simulink model "test_mdl_NI"  (R2018a)
settings: Solver=VariableStepAuto  StartTime=0.0  StopTime=10.0  RelTol=1e-3
(part 6 of 24)

== system test_mdl_NI/CAN_Signal/ECM_DIESEL PCM PCM_HEV/PowertrainData_9_0x44C ==
  in : Inport
  AutoTowActv_B_Stat : Subsystem
  AutoTowAllw_D_StatMnu : Subsystem
  GrossTrainWeight_M_Est : Subsystem
  TrailCtlPt_B_Falt : Subsystem
  Veh_V_DsplyTrailCtlSet : Subsystem
  WakeAlarm1_B_Typ : Subsystem
  WakeAlarm1_T_Rq : Subsystem
  bus_creator : BusCreator  Inputs=7
  bus_selector : BusSelector  OutputSignals=GrossTrainWeight_M_Est,AutoTowAllw_D_StatMnu,AutoTowActv_B_Stat,TrailCtlPt_B_Falt,Veh_V_DsplyTrailCtlSet,WakeAlarm1_T_Rq,WakeAlarm1_B_Typ
  out_port : Outport
  wires:
  bus_creator/1 -> out_port/1  "PowertrainData_9_0x44C"
  GrossTrainWeight_M_Est/1(out) -> bus_creator/1  "GrossTrainWeight_M_Est"
  AutoTowAllw_D_StatMnu/1(out) -> bus_creator/2  "AutoTowAllw_D_StatMnu"
  AutoTowActv_B_Stat/1(out) -> bus_creator/3  "AutoTowActv_B_Stat"
  TrailCtlPt_B_Falt/1(out) -> bus_creator/4  "TrailCtlPt_B_Falt"
  Veh_V_DsplyTrailCtlSet/1(out) -> bus_creator/5  "Veh_V_DsplyTrailCtlSet"
  WakeAlarm1_T_Rq/1(out) -> bus_creator/6  "WakeAlarm1_T_Rq"
  WakeAlarm1_B_Typ/1(out) -> bus_creator/7  "WakeAlarm1_B_Typ"
  bus_selector/1 -> GrossTrainWeight_M_Est/1(in)  "<GrossTrainWeight_M_Est>"
  bus_selector/2 -> AutoTowAllw_D_StatMnu/1(in)  "<AutoTowAllw_D_StatMnu>"
  bus_selector/3 -> AutoTowActv_B_Stat/1(in)  "<AutoTowActv_B_Stat>"
  bus_selector/4 -> TrailCtlPt_B_Falt/1(in)  "<TrailCtlPt_B_Falt>"
  bus_selector/5 -> Veh_V_DsplyTrailCtlSet/1(in)  "<Veh_V_DsplyTrailCtlSet>"
  bus_selector/6 -> WakeAlarm1_T_Rq/1(in)  "<WakeAlarm1_T_Rq>"
  bus_selector/7 -> WakeAlarm1_B_Typ/1(in)  "<WakeAlarm1_B_Typ>"
  in/1 -> bus_selector/1

== system test_mdl_NI/CAN_Signal/ECM_DIESEL PCM PCM_HEV/Powertrain_Data_4_0x424 ==
  in : Inport
  BpedDrvMsgTxt_B_Dsply : Subsystem
  FuelLvlWarn_D_ActlEng : Subsystem
  FuelLvl_Pc_DsplyEng : Subsystem
  FuelRange_L_DsplyEng : Subsystem
  RearDiffOilTeWarn_B_Rq : Subsystem
  RearDiffOil_Te_Actl : Subsystem
  SelDrvMdePt_D_Stat : Subsystem
  bus_creator : BusCreator  Inputs=7
  bus_selector : BusSelector  OutputSignals=BpedDrvMsgTxt_B_Dsply,RearDiffOil_Te_Actl,RearDiffOilTeWarn_B_Rq,FuelLvlWarn_D_ActlEng,SelDrvMdePt_D_Stat,FuelRange_L_DsplyEng,FuelLvl_Pc_DsplyEng
  out_port : Outport
  wires:
  bus_creator/1 -> out_port/1  "Powertrain_Data_4_0x424"
  BpedDrvMsgTxt_B_Dsply/1(out) -> bus_creator/1  "BpedDrvMsgTxt_B_Dsply"
  RearDiffOil_Te_Actl/1(out) -> bus_creator/2  "RearDiffOil_Te_Actl"
  RearDiffOilTeWarn_B_Rq/1(out) -> bus_creator/3  "RearDiffOilTeWarn_B_Rq"
  FuelLvlWarn_D_ActlEng/1(out) -> bus_creator/4  "FuelLvlWarn_D_ActlEng"
  SelDrvMdePt_D_Stat/1(out) -> bus_creator/5  "SelDrvMdePt_D_Stat"
  FuelRange_L_DsplyEng/1(out) -> bus_creator/6  "FuelRange_L_DsplyEng"
  FuelLvl_Pc_DsplyEng/1(out) -> bus_creator/7  "FuelLvl_Pc_DsplyEng"
  bus_selector/1 -> BpedDrvMsgTxt_B_Dsply/1(in)  "<BpedDrvMsgTxt_B_Dsply>"
  bus_selector/2 -> RearDiffOil_Te_Actl/1(in)  "<RearDiffOil_Te_Actl>"
  bus_selector/3 -> RearDiffOilTeWarn_B_Rq/1(in)  "<RearDiffOilTeWarn_B_Rq>"
  bus_selector/4 -> FuelLvlWarn_D_ActlEng/1(in)  "<FuelLvlWarn_D_ActlEng>"
  bus_selector/5 -> SelDrvMdePt_D_Stat/1(in)  "<SelDrvMdePt_D_Stat>"
  bus_selector/6 -> FuelRange_L_DsplyEng/1(in)  "<FuelRange_L_DsplyEng>"
  bus_selector/7 -> FuelLvl_Pc_DsplyEng/1(in)  "<FuelLvl_Pc_DsplyEng>"
  in/1 -> bus_selector/1

== system test_mdl_NI/CAN_Signal/ECM_DIESEL PCM PCM_HEV/Powertrain_Data_5_0x43F ==
  in : Inport
  FapLcActv_B_Stat : Subsystem
  FapLcInhbt_B_Rq : Subsystem
  FapLcMaxGrdAbrt_B_Stat : Subsystem
  FapLcMaxGrdInhbt_B_Stat : Subsystem
  FapLcObstcl_B_Stat : Subsystem
  FapLcPrchgBrk_B_Rq : Subsystem
  FapLcStopHold_B_Rq : Subsystem
  bus_creator : BusCreator  Inputs=7
  bus_selector : BusSelector  OutputSignals=FapLcActv_B_Stat,FapLcMaxGrdAbrt_B_Stat,FapLcMaxGrdInhbt_B_Stat,FapLcObstcl_B_Stat,FapLcPrchgBrk_B_Rq,FapLcStopHold_B_Rq,FapLcInhbt_B_Rq
  out_port : Outport
  wires:
  bus_creator/1 -> out_port/1  "Powertrain_Data_5_0x43F"
  FapLcActv_B_Stat/1(out) -> bus_creator/1  "FapLcActv_B_Stat"
  FapLcMaxGrdAbrt_B_Stat/1(out) -> bus_creator/2  "FapLcMaxGrdAbrt_B_Stat"
  FapLcMaxGrdInhbt_B_Stat/1(out) -> bus_creator/3  "FapLcMaxGrdInhbt_B_Stat"
  FapLcObstcl_B_Stat/1(out) -> bus_creator/4  "FapLcObstcl_B_Stat"
  FapLcPrchgBrk_B_Rq/1(out) -> bus_creator/5  "FapLcPrchgBrk_B_Rq"
  FapLcStopHold_B_Rq/1(out) -> bus_creator/6  "FapLcStopHold_B_Rq"
  FapLcInhbt_B_Rq/1(out) -> bus_creator/7  "FapLcInhbt_B_Rq"
  bus_selector/1 -> FapLcActv_B_Stat/1(in)  "<FapLcActv_B_Stat>"
  bus_selector/2 -> FapLcMaxGrdAbrt_B_Stat/1(in)  "<FapLcMaxGrdAbrt_B_Stat>"
  bus_selector/3 -> FapLcMaxGrdInhbt_B_Stat/1(in)  "<FapLcMaxGrdInhbt_B_Stat>"
  bus_selector/4 -> FapLcObstcl_B_Stat/1(in)  "<FapLcObstcl_B_Stat>"
  bus_selector/5 -> FapLcPrchgBrk_B_Rq/1(in)  "<FapLcPrchgBrk_B_Rq>"
  bus_selector/6 -> FapLcStopHold_B_Rq/1(in)  "<FapLcStopHold_B_Rq>"
  bus_selector/7 -> FapLcInhbt_B_Rq/1(in)  "<FapLcInhbt_B_Rq>"
  in/1 -> bus_selector/1

== system test_mdl_NI/CAN_Signal/ECM_DIESEL PCM PCM_HEV/Stop_Start_0x166 ==
  in : Inport
  AutoStopPtDelta_I_Est : Subsystem
  HiElPwInhbt_B_Stat : Subsystem
  OdoTripVerify_L_Actl : Subsystem
  StopStrtDrvMde_D_Indic : Subsystem
  StopStrtIODTxt_D_Rq : Subsystem
  StopStrtMsgTxt_D_Rq : Subsystem
  StopStrtStdby_D_Indic : Subsystem
  bus_creator : BusCreator  Inputs=7
  bus_selector : BusSelector  OutputSignals=AutoStopPtDelta_I_Est,HiElPwInhbt_B_Stat,StopStrtDrvMde_D_Indic,StopStrtMsgTxt_D_Rq,OdoTripVerify_L_Actl,StopStrtStdby_D_Indic,StopStrtIODTxt_D_Rq
  out_port : Outport
  wires:
  bus_creator/1 -> out_port/1  "Stop_Start_0x166"
  AutoStopPtDelta_I_Est/1(out) -> bus_creator/1  "AutoStopPtDelta_I_Est"
  HiElPwInhbt_B_Stat/1(out) -> bus_creator/2  "HiElPwInhbt_B_Stat"
  StopStrtDrvMde_D_Indic/1(out) -> bus_creator/3  "StopStrtDrvMde_D_Indic"
  StopStrtMsgTxt_D_Rq/1(out) -> bus_creator/4  "StopStrtMsgTxt_D_Rq"
  OdoTripVerify_L_Actl/1(out) -> bus_creator/5  "OdoTripVerify_L_Actl"
  StopStrtStdby_D_Indic/1(out) -> bus_creator/6  "StopStrtStdby_D_Indic"
  StopStrtIODTxt_D_Rq/1(out) -> bus_creator/7  "StopStrtIODTxt_D_Rq"
  bus_selector/1 -> AutoStopPtDelta_I_Est/1(in)  "<AutoStopPtDelta_I_Est>"
  bus_selector/2 -> HiElPwInhbt_B_Stat/1(in)  "<HiElPwInhbt_B_Stat>"
  bus_selector/3 -> StopStrtDrvMde_D_Indic/1(in)  "<StopStrtDrvMde_D_Indic>"
  bus_selector/4 -> StopStrtMsgTxt_D_Rq/1(in)  "<StopStrtMsgTxt_D_Rq>"
  bus_selector/5 -> OdoTripVerify_L_Actl/1(in)  "<OdoTripVerify_L_Actl>"
  bus_selector/6 -> StopStrtStdby_D_Indic/1(in)  "<StopStrtStdby_D_Indic>"
  bus_selector/7 -> StopStrtIODTxt_D_Rq/1(in)  "<StopStrtIODTxt_D_Rq>"
  in/1 -> bus_selector/1

== system test_mdl_NI/CAN_Signal/ECM_DIESEL PCM PCM_HEV/TesterPhysicalResPCM_0x7E8 ==
  in : Inport
  TesterPhysicalResPCM : Subsystem
  bus_creator : BusCreator  Inputs=1
  bus_selector : BusSelector  OutputSignals=TesterPhysicalResPCM
  out_port : Outport
  wires:
  bus_creator/1 -> out_port/1  "TesterPhysicalResPCM_0x7E8"
  TesterPhysicalResPCM/1(out) -> bus_creator/1  "TesterPhysicalResPCM"
  bus_selector/1 -> TesterPhysicalResPCM/1(in)  "<TesterPhysicalResPCM>"
  in/1 -> bus_selector/1

== system test_mdl_NI/CAN_Signal/ECM_DIESEL PCM PCM_HEV/TorqueDataEngFlags_0x200 ==
  in : Inport
  PrplWhlTotTqRq_No_Cnt : Subsystem
  PrplWhlTotTqRq_No_Cs : Subsystem
  PrplWhlTot_Tq_LimMn : Subsystem
  PrplWhlTot_Tq_Rq : Subsystem
  PtDrvMde_D_Stat : Subsystem
  bus_creator : BusCreator  Inputs=5
  bus_selector : BusSelector  OutputSignals=PrplWhlTot_Tq_LimMn,PrplWhlTot_Tq_Rq,PtDrvMde_D_Stat,PrplWhlTotTqRq_No_Cnt,PrplWhlTotTqRq_No_Cs
  out_port : Outport
  wires:
  bus_creator/1 -> out_port/1  "TorqueDataEngFlags_0x200"
  PrplWhlTot_Tq_LimMn/1(out) -> bus_creator/1  "PrplWhlTot_Tq_LimMn"
  PrplWhlTot_Tq_Rq/1(out) -> bus_creator/2  "PrplWhlTot_Tq_Rq"
  PtDrvMde_D_Stat/1(out) -> bus_creator/3  "PtDrvMde_D_Stat"
  PrplWhlTotTqRq_No_Cnt/1(out) -> bus_creator/4  "PrplWhlTotTqRq_No_Cnt"
  PrplWhlTotTqRq_No_Cs/1(out) -> bus_creator/5  "PrplWhlTotTqRq_No_Cs"
  bus_selector/1 -> PrplWhlTot_Tq_LimMn/1(in)  "<PrplWhlTot_Tq_LimMn>"
  bus_selector/2 -> PrplWhlTot_Tq_Rq/1(in)  "<PrplWhlTot_Tq_Rq>"
  bus_selector/3 -> PtDrvMde_D_Stat/1(in)  "<PtDrvMde_D_Stat>"
  bus_selector/4 -> PrplWhlTotTqRq_No_Cnt/1(in)  "<PrplWhlTotTqRq_No_Cnt>"
  bus_selector/5 -> PrplWhlTotTqRq_No_Cs/1(in)  "<PrplWhlTotTqRq_No_Cs>"
  in/1 -> bus_selector/1

== system test_mdl_NI/CAN_Signal/ECM_DIESEL PCM PCM_HEV/TransGearData ==
  in : Inport
  GboxOil_Te_Actl : Subsystem
  GearLvrPos_D_Actl : Subsystem
  SelDrvMdeSwtch_D_Stat3 : Subsystem
  TrnShifActv_B_Actl : Subsystem
  TrnSrvcRqd_B_Rq : Subsystem
  bus_creator : BusCreator  Inputs=5
  bus_selector : BusSelector  OutputSignals=GboxOil_Te_Actl,GearLvrPos_D_Actl,SelDrvMdeSwtch_D_Stat3,TrnShifActv_B_Actl,TrnSrvcRqd_B_Rq
  out_port : Outport
  wires:
  bus_creator/1 -> out_port/1  "TransGearData"
  GboxOil_Te_Actl/1(out) -> bus_creator/1  "GboxOil_Te_Actl"
  GearLvrPos_D_Actl/1(out) -> bus_creator/2  "GearLvrPos_D_Actl"
  SelDrvMdeSwtch_D_Stat3/1(out) -> bus_creator/3  "SelDrvMdeSwtch_D_Stat3"
  TrnShifActv_B_Actl/1(out) -> bus_creator/4  "TrnShifActv_B_Actl"
  TrnSrvcRqd_B_Rq/1(out) -> bus_creator/5  "TrnSrvcRqd_B_Rq"
  bus_selector/1 -> GboxOil_Te_Actl/1(in)  "<GboxOil_Te_Actl>"
  bus_selector/2 -> GearLvrPos_D_Actl/1(in)  "<GearLvrPos_D_Actl>"
  bus_selector/3 -> SelDrvMdeSwtch_D_Stat3/1(in)  "<SelDrvMdeSwtch_D_Stat3>"
  bus_selector/4 -> TrnShifActv_B_Actl/1(in)  "<TrnShifActv_B_Actl>"
  bus_selector/5 -> TrnSrvcRqd_B_Rq/1(in)  "<TrnSrvcRqd_B_Rq>"
  in/1 -> bus_selector/1

== system test_mdl_NI/CAN_Signal/ECM_DIESEL PCM PCM_HEV/VehicleOperatingModes_0x167 ==
  in : Inport
  ElPw_D_Stat : Subsystem
  ElPw_D_StatStrtStop : Subsystem
  Eng_D_Stat : Subsystem
  PlgActvArb_B_Actl : Subsystem
  PrplWhlRgenMn_Tq_Actl : Subsystem
  PrplWhlTot2_Tq_Actl : Subsystem
  PwPckTq_D_Stat : Subsystem
  TrnAinTq_D_Qf : Subsystem
  TrnAin_Tq_Actl : Subsystem
  bus_creator : BusCreator  Inputs=9
  bus_selector : BusSelector  OutputSignals=Eng_D_Stat,PwPckTq_D_Stat,ElPw_D_Stat,PlgActvArb_B_Actl,PrplWhlTot2_Tq_Actl,ElPw_D_StatStrtStop,PrplWhlRgenMn_Tq_Actl,TrnAinTq_D_Qf,TrnAin_Tq_Actl
  out_port : Outport
  wires:
  bus_creator/1 -> out_port/1  "VehicleOperatingModes_0x167"
  Eng_D_Stat/1(out) -> bus_creator/1  "Eng_D_Stat"
  PwPckTq_D_Stat/1(out) -> bus_creator/2  "PwPckTq_D_Stat"
  ElPw_D_Stat/1(out) -> bus_creator/3  "ElPw_D_Stat"
  PlgActvArb_B_Actl/1(out) -> bus_creator/4  "PlgActvArb_B_Actl"
  PrplWhlTot2_Tq_Actl/1(out) -> bus_creator/5  "PrplWhlTot2_Tq_Actl"
  ElPw_D_StatStrtStop/1(out) -> bus_creator/6  "ElPw_D_StatStrtStop"
  PrplWhlRgenMn_Tq_Actl/1(out) -> bus_creator/7  "PrplWhlRgenMn_Tq_Actl"
  TrnAinTq_D_Qf/1(out) -> bus_creator/8  "TrnAinTq_D_Qf"
  TrnAin_Tq_Actl/1(out) -> bus_creator/9  "TrnAin_Tq_Actl"
  bus_selector/1 -> Eng_D_Stat/1(in)  "<Eng_D_Stat>"
  bus_selector/2 -> PwPckTq_D_Stat/1(in)  "<PwPckTq_D_Stat>"
  bus_selector/3 -> ElPw_D_Stat/1(in)  "<ElPw_D_Stat>"
  bus_selector/4 -> PlgActvArb_B_Actl/1(in)  "<PlgActvArb_B_Actl>"
  bus_selector/5 -> PrplWhlTot2_Tq_Actl/1(in)  "<PrplWhlTot2_Tq_Actl>"
  bus_selector/6 -> ElPw_D_StatStrtStop/1(in)  "<ElPw_D_StatStrtStop>"
  bus_selector/7 -> PrplWhlRgenMn_Tq_Actl/1(in)  "<PrplWhlRgenMn_Tq_Actl>"
  bus_selector/8 -> TrnAinTq_D_Qf/1(in)  "<TrnAinTq_D_Qf>"
  bus_selector/9 -> TrnAin_Tq_Actl/1(in)  "<TrnAin_Tq_Actl>"
  in/1 -> bus_selector/1

== system test_mdl_NI/CAN_Signal/GWM/GSM ==
  in : Inport
  Gear_Shift_by_Wire_2_FD1_168 : Subsystem
  Gear_Shift_by_Wire_FD1_5A : Subsystem
  bus_creator : BusCreator  Inputs=2
  bus_selector : BusSelector  OutputSignals=Gear_Shift_by_Wire_2_FD1_168,Gear_Shift_by_Wire_FD1_5A
  out_port : Outport
  wires:
  bus_creator/1 -> out_port/1  "GSM"
  Gear_Shift_by_Wire_2_FD1_168/1(out_port) -> bus_creator/1  "Gear_Shift_by_Wire_2_FD1_168"
  Gear_Shift_by_Wire_FD1_5A/1(out_port) -> bus_creator/2  "Gear_Shift_by_Wire_FD1_5A"
  bus_selector/1 -> Gear_Shift_by_Wire_2_FD1_168/1(in)  "<Gear_Shift_by_Wire_2_FD1_168>"
  bus_selector/2 -> Gear_Shift_by_Wire_FD1_5A/1(in)  "<Gear_Shift_by_Wire_FD1_5A>"
  in/1 -> bus_selector/1

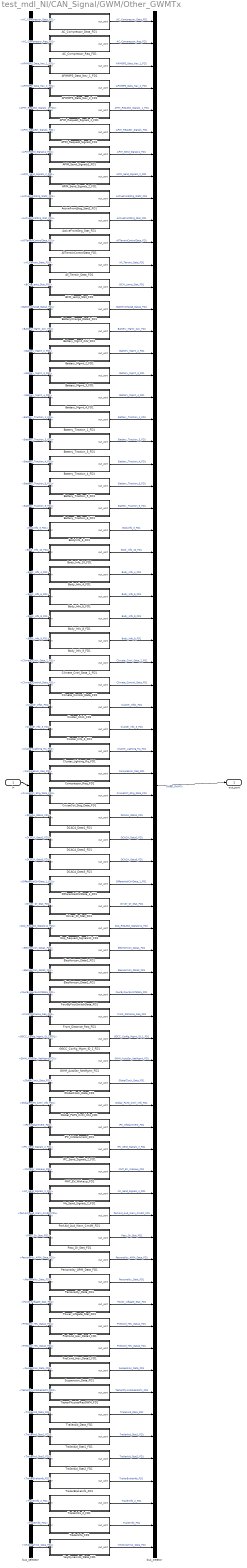
== system test_mdl_NI/CAN_Signal/GWM/Other_GWMTx ==
  in : Inport
  AC_Compressor_Data_FD1 : Subsystem
  AC_Compressor_Req_FD1 : Subsystem
  APIMGPS_Data_Nav_1_FD1 : Subsystem
  APIMGPS_Data_Nav_2_FD1 : Subsystem
  APIM_Request_Signals_1_FD1 : Subsystem
  APIM_Request_Signals_FD1 : Subsystem
  APIM_Send_Signals1_FD1 : Subsystem
  APIM_Send_Signals_2_FD1 : Subsystem
  ActiveFrontStrg_Stat2_FD1 : Subsystem
  ActiveFrontStrg_Stat_FD1 : Subsystem
  AllTerrainControlData_FD1 : Subsystem
  All_Terrain_Data_FD1 : Subsystem
  BCM_Lamp_Stat_FD1 : Subsystem
  BatteryCharge_Data2_FD1 : Subsystem
  Battery_Mgmt_24V_FD1 : Subsystem
  Battery_Mgmt_2_FD1 : Subsystem
  Battery_Mgmt_3_FD1 : Subsystem
  Battery_Mgmt_4_FD1 : Subsystem
  Battery_Traction_1_FD1 : Subsystem
  Battery_Traction_3_FD1 : Subsystem
  Battery_Traction_4_FD1 : Subsystem
  Battery_Traction_5_FD1 : Subsystem
  Battery_Traction_6_FD1 : Subsystem
  BodyInfo_3_FD1 : Subsystem
  Body_Info_10_FD1 : Subsystem
  Body_Info_4_FD1 : Subsystem
  Body_Info_6_FD1 : Subsystem
  Body_Info_8_FD1 : Subsystem
  Body_Info_9_FD1 : Subsystem
  Climate_Cntrl_Data_2_FD1 : Subsystem
  Climate_Control_Data_FD1 : Subsystem
  Cluster_Info1_FD1 : Subsystem
  Cluster_Info_3_FD1 : Subsystem
  Cluster_Lighting_Rq_FD1 : Subsystem
  Compressor_Req_FD1 : Subsystem
  CruiseCtrl_Strg_Data_FD1 : Subsystem
  DCACA_Data1_FD1 : Subsystem
  DCACA_Data2_FD1 : Subsystem
  DCACA_Data3_FD1 : Subsystem
  DifferentialCtrlData_1_FD1 : Subsystem
  Driver_Dr_Stat_FD1 : Subsystem
  Dsp_Request_Signals11_FD1 : Subsystem
  ElecHorizon_Data1_FD1 : Subsystem
  ElecHorizon_Data2_FD1 : Subsystem
  FourByFourSwitchData_FD1 : Subsystem
  Front_Distance_Req_FD1 : Subsystem
  GGCC_Config_Mgmt_ID_1_FD1 : Subsystem
  GWM_AutoSar_NetMgmt_FD1 : Subsystem
  GlobalClock_Data_FD1 : Subsystem
  Global_PATS_Cntrl_Info_FD1 : Subsystem
  IPC_Infotainment_FD1 : Subsystem
  IPC_Send_Signals_2_FD1 : Subsystem
  MHT_EV_Wakeup_FD1 : Subsystem
  Mc_Send_Signals_2_FD1 : Subsystem
  ParkAid_Aud_Warn_CmdM_FD1 : Subsystem
  Pass_Dr_Stat_FD1 : Subsystem
  Personality_APIM_Data_FD1 : Subsystem
  Personality_Data_FD1 : Subsystem
  Power_Liftgate_Stat_FD1 : Subsystem
  PreCond_Hev_Data1_FD1 : Subsystem
  PreCond_Hev_Data2_FD1 : Subsystem
  Suspension_Data_FD1 : Subsystem
  TesterPhysicalResGWM_FD1 : Subsystem
  TrailerAid_Data_FD1 : Subsystem
  TrailerAid_Stat1_FD1 : Subsystem
  TrailerAid_Stat2_FD1 : Subsystem
  TrailerBrakeInfo_FD1 : Subsystem
  TrailerInfo_2_FD1 : Subsystem
  TrailerInfo_FD1 : Subsystem
  VeyDynamics_Data_FD1 : Subsystem
  bus_creator : BusCreator  Inputs=70
  bus_selector : BusSelector  OutputSignals=AC_Compressor_Data_FD1,AC_Compressor_Req_FD1,APIMGPS_Data_Nav_1_FD1,APIMGPS_Data_Nav_2_FD1,APIM_Request_Signals_1_FD1,APIM_Request_Signals_FD1,APIM_Send_Signals1_FD1,APIM_Send_Signals_2_FD1,ActiveFrontStrg_Stat2_FD1,ActiveFrontStrg_Stat_FD1,AllTerrainControlData_FD1,All_Terrain_Data_FD1,BCM_Lamp_Stat_FD1,BatteryCharge_Data2_FD1,Battery_Mgmt_24V_FD1,Battery_Mgmt_2_FD1,Battery_Mgmt_3_FD1,Battery_Mgmt_4_FD1,Battery_Traction_1_FD1,Battery_Traction_3_FD1,Battery_Traction_4_FD1,Battery_Traction_5_FD1,Battery_Traction_6_FD1,BodyInfo_3_FD1,Body_Info_10_FD1,Body_Info_4_FD1,Body_Info_6_FD1,Body_Info_8_FD1,Body_Info_9_FD1,Climate_Cntrl_Data_2_FD1,Climate_Control_Data_FD1,Cluster_Info1_FD1,Cluster_Info_3_FD1,Cluster_Lighting_Rq_FD1,Compressor_Req_FD1,CruiseCtrl_Strg_Data_FD1,DCACA_Data1_FD1,DCACA_Data2_FD1,DCACA_Data3_FD1,DifferentialCtrlData_1_FD1,Driver_Dr_Stat_FD1,Dsp_Request_Signals11_FD1,ElecHorizon_Data1_FD1,ElecHorizon_Data2_FD1,FourByFourSwitchData_FD1,Front_Distance_Req_FD1,GGCC_Config_Mgmt_ID_1_FD1,GWM_AutoSar_NetMgmt_FD1,GlobalClock_Data_FD1,Global_PATS_Cntrl_Info_FD1,IPC_Infotainment_FD1,IPC_Send_Signals_2_FD1,MHT_EV_Wakeup_FD1,Mc_Send_Signals_2_FD1,ParkAid_Aud_Warn_CmdM_FD1,Pass_Dr_Stat_FD1,Personality_APIM_Data_FD1,Personality_Data_FD1,Power_Liftgate_Stat_FD1,PreCond_Hev_Data1_FD1,PreCond_Hev_Data2_FD1,Suspension_Data_FD1,TesterPhysicalResGWM_FD1,TrailerAid_Data_FD1,TrailerAid_Stat1_FD1,TrailerAid_Stat2_FD1,TrailerBrakeInfo_FD1,TrailerInfo_2_FD1,TrailerInfo_FD1,VeyDynamics_Data_FD1
  out_port : Outport
  wires:
  bus_creator/1 -> out_port/1  "Other_GWMTx"
  AC_Compressor_Data_FD1/1(out_port) -> bus_creator/1  "AC_Compressor_Data_FD1"
  AC_Compressor_Req_FD1/1(out_port) -> bus_creator/2  "AC_Compressor_Req_FD1"
  APIMGPS_Data_Nav_1_FD1/1(out_port) -> bus_creator/3  "APIMGPS_Data_Nav_1_FD1"
  APIMGPS_Data_Nav_2_FD1/1(out_port) -> bus_creator/4  "APIMGPS_Data_Nav_2_FD1"
  APIM_Request_Signals_1_FD1/1(out_port) -> bus_creator/5  "APIM_Request_Signals_1_FD1"
  APIM_Request_Signals_FD1/1(out_port) -> bus_creator/6  "APIM_Request_Signals_FD1"
  APIM_Send_Signals1_FD1/1(out_port) -> bus_creator/7  "APIM_Send_Signals1_FD1"
  APIM_Send_Signals_2_FD1/1(out_port) -> bus_creator/8  "APIM_Send_Signals_2_FD1"
  ActiveFrontStrg_Stat2_FD1/1(out_port) -> bus_creator/9  "ActiveFrontStrg_Stat2_FD1"
  ActiveFrontStrg_Stat_FD1/1(out_port) -> bus_creator/10  "ActiveFrontStrg_Stat_FD1"
  AllTerrainControlData_FD1/1(out_port) -> bus_creator/11  "AllTerrainControlData_FD1"
  All_Terrain_Data_FD1/1(out_port) -> bus_creator/12  "All_Terrain_Data_FD1"
  BCM_Lamp_Stat_FD1/1(out_port) -> bus_creator/13  "BCM_Lamp_Stat_FD1"
  BatteryCharge_Data2_FD1/1(out_port) -> bus_creator/14  "BatteryCharge_Data2_FD1"
  Battery_Mgmt_24V_FD1/1(out_port) -> bus_creator/15  "Battery_Mgmt_24V_FD1"
  Battery_Mgmt_2_FD1/1(out_port) -> bus_creator/16  "Battery_Mgmt_2_FD1"
  Battery_Mgmt_3_FD1/1(out_port) -> bus_creator/17  "Battery_Mgmt_3_FD1"
  Battery_Mgmt_4_FD1/1(out_port) -> bus_creator/18  "Battery_Mgmt_4_FD1"
  Battery_Traction_1_FD1/1(out_port) -> bus_creator/19  "Battery_Traction_1_FD1"
  Battery_Traction_3_FD1/1(out_port) -> bus_creator/20  "Battery_Traction_3_FD1"
  Battery_Traction_4_FD1/1(out_port) -> bus_creator/21  "Battery_Traction_4_FD1"
  Battery_Traction_5_FD1/1(out_port) -> bus_creator/22  "Battery_Traction_5_FD1"
  Battery_Traction_6_FD1/1(out_port) -> bus_creator/23  "Battery_Traction_6_FD1"
  BodyInfo_3_FD1/1(out_port) -> bus_creator/24  "BodyInfo_3_FD1"
  Body_Info_10_FD1/1(out_port) -> bus_creator/25  "Body_Info_10_FD1"
  Body_Info_4_FD1/1(out_port) -> bus_creator/26  "Body_Info_4_FD1"
  Body_Info_6_FD1/1(out_port) -> bus_creator/27  "Body_Info_6_FD1"
  Body_Info_8_FD1/1(out_port) -> bus_creator/28  "Body_Info_8_FD1"
  Body_Info_9_FD1/1(out_port) -> bus_creator/29  "Body_Info_9_FD1"
  Climate_Cntrl_Data_2_FD1/1(out_port) -> bus_creator/30  "Climate_Cntrl_Data_2_FD1"
  Climate_Control_Data_FD1/1(out_port) -> bus_creator/31  "Climate_Control_Data_FD1"
  Cluster_Info1_FD1/1(out_port) -> bus_creator/32  "Cluster_Info1_FD1"
  Cluster_Info_3_FD1/1(out_port) -> bus_creator/33  "Cluster_Info_3_FD1"
  Cluster_Lighting_Rq_FD1/1(out_port) -> bus_creator/34  "Cluster_Lighting_Rq_FD1"
  Compressor_Req_FD1/1(out_port) -> bus_creator/35  "Compressor_Req_FD1"
  CruiseCtrl_Strg_Data_FD1/1(out_port) -> bus_creator/36  "CruiseCtrl_Strg_Data_FD1"
  DCACA_Data1_FD1/1(out_port) -> bus_creator/37  "DCACA_Data1_FD1"
  DCACA_Data2_FD1/1(out_port) -> bus_creator/38  "DCACA_Data2_FD1"
  DCACA_Data3_FD1/1(out_port) -> bus_creator/39  "DCACA_Data3_FD1"
  DifferentialCtrlData_1_FD1/1(out_port) -> bus_creator/40  "DifferentialCtrlData_1_FD1"
  Driver_Dr_Stat_FD1/1(out_port) -> bus_creator/41  "Driver_Dr_Stat_FD1"
  Dsp_Request_Signals11_FD1/1(out_port) -> bus_creator/42  "Dsp_Request_Signals11_FD1"
  ElecHorizon_Data1_FD1/1(out_port) -> bus_creator/43  "ElecHorizon_Data1_FD1"
  ElecHorizon_Data2_FD1/1(out_port) -> bus_creator/44  "ElecHorizon_Data2_FD1"
  FourByFourSwitchData_FD1/1(out_port) -> bus_creator/45  "FourByFourSwitchData_FD1"
  Front_Distance_Req_FD1/1(out_port) -> bus_creator/46  "Front_Distance_Req_FD1"
  GGCC_Config_Mgmt_ID_1_FD1/1(out_port) -> bus_creator/47  "GGCC_Config_Mgmt_ID_1_FD1"
  GWM_AutoSar_NetMgmt_FD1/1(out_port) -> bus_creator/48  "GWM_AutoSar_NetMgmt_FD1"
  GlobalClock_Data_FD1/1(out_port) -> bus_creator/49  "GlobalClock_Data_FD1"
  Global_PATS_Cntrl_Info_FD1/1(out_port) -> bus_creator/50  "Global_PATS_Cntrl_Info_FD1"
  IPC_Infotainment_FD1/1(out_port) -> bus_creator/51  "IPC_Infotainment_FD1"
  IPC_Send_Signals_2_FD1/1(out_port) -> bus_creator/52  "IPC_Send_Signals_2_FD1"
  MHT_EV_Wakeup_FD1/1(out_port) -> bus_creator/53  "MHT_EV_Wakeup_FD1"
  Mc_Send_Signals_2_FD1/1(out_port) -> bus_creator/54  "Mc_Send_Signals_2_FD1"
  ParkAid_Aud_Warn_CmdM_FD1/1(out_port) -> bus_creator/55  "ParkAid_Aud_Warn_CmdM_FD1"
  Pass_Dr_Stat_FD1/1(out_port) -> bus_creator/56  "Pass_Dr_Stat_FD1"
  Personality_APIM_Data_FD1/1(out_port) -> bus_creator/57  "Personality_APIM_Data_FD1"
  Personality_Data_FD1/1(out_port) -> bus_creator/58  "Personality_Data_FD1"
  Power_Liftgate_Stat_FD1/1(out_port) -> bus_creator/59  "Power_Liftgate_Stat_FD1"
  PreCond_Hev_Data1_FD1/1(out_port) -> bus_creator/60  "PreCond_Hev_Data1_FD1"
  PreCond_Hev_Data2_FD1/1(out_port) -> bus_creator/61  "PreCond_Hev_Data2_FD1"
  Suspension_Data_FD1/1(out_port) -> bus_creator/62  "Suspension_Data_FD1"
  TesterPhysicalResGWM_FD1/1(out_port) -> bus_creator/63  "TesterPhysicalResGWM_FD1"
  TrailerAid_Data_FD1/1(out_port) -> bus_creator/64  "TrailerAid_Data_FD1"
  TrailerAid_Stat1_FD1/1(out_port) -> bus_creator/65  "TrailerAid_Stat1_FD1"
  TrailerAid_Stat2_FD1/1(out_port) -> bus_creator/66  "TrailerAid_Stat2_FD1"
  TrailerBrakeInfo_FD1/1(out_port) -> bus_creator/67  "TrailerBrakeInfo_FD1"
  TrailerInfo_2_FD1/1(out_port) -> bus_creator/68  "TrailerInfo_2_FD1"
  TrailerInfo_FD1/1(out_port) -> bus_creator/69  "TrailerInfo_FD1"
  VeyDynamics_Data_FD1/1(out_port) -> bus_creator/70  "VeyDynamics_Data_FD1"
  bus_selector/1 -> AC_Compressor_Data_FD1/1(in)  "<AC_Compressor_Data_FD1>"
  bus_selector/2 -> AC_Compressor_Req_FD1/1(in)  "<AC_Compressor_Req_FD1>"
  bus_selector/3 -> APIMGPS_Data_Nav_1_FD1/1(in)  "<APIMGPS_Data_Nav_1_FD1>"
  bus_selector/4 -> APIMGPS_Data_Nav_2_FD1/1(in)  "<APIMGPS_Data_Nav_2_FD1>"
  bus_selector/5 -> APIM_Request_Signals_1_FD1/1(in)  "<APIM_Request_Signals_1_FD1>"
  bus_selector/6 -> APIM_Request_Signals_FD1/1(in)  "<APIM_Request_Signals_FD1>"
  bus_selector/7 -> APIM_Send_Signals1_FD1/1(in)  "<APIM_Send_Signals1_FD1>"
  bus_selector/8 -> APIM_Send_Signals_2_FD1/1(in)  "<APIM_Send_Signals_2_FD1>"
  bus_selector/9 -> ActiveFrontStrg_Stat2_FD1/1(in)  "<ActiveFrontStrg_Stat2_FD1>"
  bus_selector/10 -> ActiveFrontStrg_Stat_FD1/1(in)  "<ActiveFrontStrg_Stat_FD1>"
  bus_selector/11 -> AllTerrainControlData_FD1/1(in)  "<AllTerrainControlData_FD1>"
  bus_selector/12 -> All_Terrain_Data_FD1/1(in)  "<All_Terrain_Data_FD1>"
  bus_selector/13 -> BCM_Lamp_Stat_FD1/1(in)  "<BCM_Lamp_Stat_FD1>"
  bus_selector/14 -> BatteryCharge_Data2_FD1/1(in)  "<BatteryCharge_Data2_FD1>"
  bus_selector/15 -> Battery_Mgmt_24V_FD1/1(in)  "<Battery_Mgmt_24V_FD1>"
  bus_selector/16 -> Battery_Mgmt_2_FD1/1(in)  "<Battery_Mgmt_2_FD1>"
  bus_selector/17 -> Battery_Mgmt_3_FD1/1(in)  "<Battery_Mgmt_3_FD1>"
  bus_selector/18 -> Battery_Mgmt_4_FD1/1(in)  "<Battery_Mgmt_4_FD1>"
  bus_selector/19 -> Battery_Traction_1_FD1/1(in)  "<Battery_Traction_1_FD1>"
  bus_selector/20 -> Battery_Traction_3_FD1/1(in)  "<Battery_Traction_3_FD1>"
  bus_selector/21 -> Battery_Traction_4_FD1/1(in)  "<Battery_Traction_4_FD1>"
  bus_selector/22 -> Battery_Traction_5_FD1/1(in)  "<Battery_Traction_5_FD1>"
  bus_selector/23 -> Battery_Traction_6_FD1/1(in)  "<Battery_Traction_6_FD1>"
  bus_selector/24 -> BodyInfo_3_FD1/1(in)  "<BodyInfo_3_FD1>"
  bus_selector/25 -> Body_Info_10_FD1/1(in)  "<Body_Info_10_FD1>"
  bus_selector/26 -> Body_Info_4_FD1/1(in)  "<Body_Info_4_FD1>"
  bus_selector/27 -> Body_Info_6_FD1/1(in)  "<Body_Info_6_FD1>"
  bus_selector/28 -> Body_Info_8_FD1/1(in)  "<Body_Info_8_FD1>"
  bus_selector/29 -> Body_Info_9_FD1/1(in)  "<Body_Info_9_FD1>"
  bus_selector/30 -> Climate_Cntrl_Data_2_FD1/1(in)  "<Climate_Cntrl_Data_2_FD1>"
  bus_selector/31 -> Climate_Control_Data_FD1/1(in)  "<Climate_Control_Data_FD1>"
  bus_selector/32 -> Cluster_Info1_FD1/1(in)  "<Cluster_Info1_FD1>"
  bus_selector/33 -> Cluster_Info_3_FD1/1(in)  "<Cluster_Info_3_FD1>"
  bus_selector/34 -> Cluster_Lighting_Rq_FD1/1(in)  "<Cluster_Lighting_Rq_FD1>"
  bus_selector/35 -> Compressor_Req_FD1/1(in)  "<Compressor_Req_FD1>"
  bus_selector/36 -> CruiseCtrl_Strg_Data_FD1/1(in)  "<CruiseCtrl_Strg_Data_FD1>"
  bus_selector/37 -> DCACA_Data1_FD1/1(in)  "<DCACA_Data1_FD1>"
  bus_selector/38 -> DCACA_Data2_FD1/1(in)  "<DCACA_Data2_FD1>"
  bus_selector/39 -> DCACA_Data3_FD1/1(in)  "<DCACA_Data3_FD1>"
  bus_selector/40 -> DifferentialCtrlData_1_FD1/1(in)  "<DifferentialCtrlData_1_FD1>"
  bus_selector/41 -> Driver_Dr_Stat_FD1/1(in)  "<Driver_Dr_Stat_FD1>"
  bus_selector/42 -> Dsp_Request_Signals11_FD1/1(in)  "<Dsp_Request_Signals11_FD1>"
  bus_selector/43 -> ElecHorizon_Data1_FD1/1(in)  "<ElecHorizon_Data1_FD1>"
  bus_selector/44 -> ElecHorizon_Data2_FD1/1(in)  "<ElecHorizon_Data2_FD1>"
  bus_selector/45 -> FourByFourSwitchData_FD1/1(in)  "<FourByFourSwitchData_FD1>"
  bus_selector/46 -> Front_Distance_Req_FD1/1(in)  "<Front_Distance_Req_FD1>"
  bus_selector/47 -> GGCC_Config_Mgmt_ID_1_FD1/1(in)  "<GGCC_Config_Mgmt_ID_1_FD1>"
  bus_selector/48 -> GWM_AutoSar_NetMgmt_FD1/1(in)  "<GWM_AutoSar_NetMgmt_FD1>"
  bus_selector/49 -> GlobalClock_Data_FD1/1(in)  "<GlobalClock_Data_FD1>"
  bus_selector/50 -> Global_PATS_Cntrl_Info_FD1/1(in)  "<Global_PATS_Cntrl_Info_FD1>"
  bus_selector/51 -> IPC_Infotainment_FD1/1(in)  "<IPC_Infotainment_FD1>"
  bus_selector/52 -> IPC_Send_Signals_2_FD1/1(in)  "<IPC_Send_Signals_2_FD1>"
  bus_selector/53 -> MHT_EV_Wakeup_FD1/1(in)  "<MHT_EV_Wakeup_FD1>"
  bus_selector/54 -> Mc_Send_Signals_2_FD1/1(in)  "<Mc_Send_Signals_2_FD1>"
  bus_selector/55 -> ParkAid_Aud_Warn_CmdM_FD1/1(in)  "<ParkAid_Aud_Warn_CmdM_FD1>"
  bus_selector/56 -> Pass_Dr_Stat_FD1/1(in)  "<Pass_Dr_Stat_FD1>"
  bus_selector/57 -> Personality_APIM_Data_FD1/1(in)  "<Personality_APIM_Data_FD1>"
  bus_selector/58 -> Personality_Data_FD1/1(in)  "<Personality_Data_FD1>"
  bus_selector/59 -> Power_Liftgate_Stat_FD1/1(in)  "<Power_Liftgate_Stat_FD1>"
  bus_selector/60 -> PreCond_Hev_Data1_FD1/1(in)  "<PreCond_Hev_Data1_FD1>"
  bus_selector/61 -> PreCond_Hev_Data2_FD1/1(in)  "<PreCond_Hev_Data2_FD1>"
  bus_selector/62 -> Suspension_Data_FD1/1(in)  "<Suspension_Data_FD1>"
  bus_selector/63 -> TesterPhysicalResGWM_FD1/1(in)  "<TesterPhysicalResGWM_FD1>"
  bus_selector/64 -> TrailerAid_Data_FD1/1(in)  "<TrailerAid_Data_FD1>"
  bus_selector/65 -> TrailerAid_Stat1_FD1/1(in)  "<TrailerAid_Stat1_FD1>"
  bus_selector/66 -> TrailerAid_Stat2_FD1/1(in)  "<TrailerAid_Stat2_FD1>"
  bus_selector/67 -> TrailerBrakeInfo_FD1/1(in)  "<TrailerBrakeInfo_FD1>"
  bus_selector/68 -> TrailerInfo_2_FD1/1(in)  "<TrailerInfo_2_FD1>"
  bus_selector/69 -> TrailerInfo_FD1/1(in)  "<TrailerInfo_FD1>"
  bus_selector/70 -> VeyDynamics_Data_FD1/1(in)  "<VeyDynamics_Data_FD1>"
  in/1 -> bus_selector/1

== system test_mdl_NI/CAN_Signal/GWM/RCM ==
  in : Inport
  RCMSerialNumber_FD1_454 : Subsystem
  RCMStatusMessage2_FD1_4C : Subsystem
  bus_creator : BusCreator  Inputs=2
  bus_selector : BusSelector  OutputSignals=RCMStatusMessage2_FD1_4C,RCMSerialNumber_FD1_454
  out_port : Outport
  wires:
  bus_creator/1 -> out_port/1  "RCM"
  RCMStatusMessage2_FD1_4C/1(out_port) -> bus_creator/1  "RCMStatusMessage2_FD1_4C"
  RCMSerialNumber_FD1_454/1(out_port) -> bus_creator/2  "RCMSerialNumber_FD1_454"
  bus_selector/1 -> RCMStatusMessage2_FD1_4C/1(in)  "<RCMStatusMessage2_FD1_4C>"
  bus_selector/2 -> RCMSerialNumber_FD1_454/1(in)  "<RCMSerialNumber_FD1_454>"
  in/1 -> bus_selector/1

== system test_mdl_NI/CAN_Signal/GWM/SCCM ==
  in : Inport
  Steering_Data_FD1_83 : Subsystem
  Steering_Wheel_Data2_FD1_81 : Subsystem
  bus_creator : BusCreator  Inputs=2
  bus_selector : BusSelector  OutputSignals=Steering_Data_FD1_83,Steering_Wheel_Data2_FD1_81
  out_port : Outport
  wires:
  bus_creator/1 -> out_port/1  "SCCM"
  Steering_Data_FD1_83/1(out_port) -> bus_creator/1  "Steering_Data_FD1_83"
  Steering_Wheel_Data2_FD1_81/1(out_port) -> bus_creator/2  "Steering_Wheel_Data2_FD1_81"
  bus_selector/1 -> Steering_Data_FD1_83/1(in)  "<Steering_Data_FD1_83>"
  bus_selector/2 -> Steering_Wheel_Data2_FD1_81/1(in)  "<Steering_Wheel_Data2_FD1_81>"
  in/1 -> bus_selector/1

== system test_mdl_NI/CAN_Signal/GWM/Tester_AutoSar ==
  in : Inport
  GWM_AutoSar_NetMgmt_FD1 : Subsystem
  TesterPhysicalResGWM_FD1 : Subsystem
  bus_creator : BusCreator  Inputs=2
  bus_selector : BusSelector  OutputSignals=GWM_AutoSar_NetMgmt_FD1,TesterPhysicalResGWM_FD1
  out_port : Outport
  wires:
  bus_creator/1 -> out_port/1  "Tester_AutoSar"
  GWM_AutoSar_NetMgmt_FD1/1(out_port) -> bus_creator/1  "GWM_AutoSar_NetMgmt_FD1"
  TesterPhysicalResGWM_FD1/1(out_port) -> bus_creator/2  "TesterPhysicalResGWM_FD1"
  bus_selector/1 -> GWM_AutoSar_NetMgmt_FD1/1(in)  "<GWM_AutoSar_NetMgmt_FD1>"
  bus_selector/2 -> TesterPhysicalResGWM_FD1/1(in)  "<TesterPhysicalResGWM_FD1>"
  in/1 -> bus_selector/1

== system test_mdl_NI/CAN_Signal/PSCM/EPAS_INFO_0x82 ==
  in : Inport
  DrvSteActv_B_Stat : Subsystem
  DrvSte_Tq_Actl : Subsystem
  EPAS_Failure : Subsystem
  SAPPAngleControlStat1 : Subsystem
  SAPPAngleControlStat2 : Subsystem
  SAPPAngleControlStat3 : Subsystem
  SAPPAngleControlStat4 : Subsystem
  SAPPAngleControlStat5 : Subsystem
  SAPPAngleControlStat6 : Subsystem
  SteMdule_D_Stat : Subsystem
  SteMdule_I_Est : Subsystem
  SteMdule_U_Meas : Subsystem
  SteeringColumnTorque : Subsystem
  TrlrHitchLamp_D_Rqst : Subsystem
  VehVTrlrAid_B_Rq : Subsystem
  Veh_V_RqMxTrlrAid : Subsystem
  bus_creator : BusCreator  Inputs=16
  bus_selector : BusSelector  OutputSignals=SteeringColumnTorque,SAPPAngleControlStat6,SAPPAngleControlStat5,SAPPAngleControlStat4,SAPPAngleControlStat3,SAPPAngleControlStat2,DrvSteActv_B_Stat,EPAS_Failure,SAPPAngleControlStat1,SteMdule_I_Est,VehVTrlrAid_B_Rq,TrlrHitchLamp_D_Rqst,SteMdule_U_Meas,DrvSte_Tq_Actl,SteMdule_D_Stat,Veh_V_RqMxTrlrAid
  out_port : Outport
  wires:
  bus_creator/1 -> out_port/1  "EPAS_INFO_0x82"
  SteeringColumnTorque/1(out) -> bus_creator/1  "SteeringColumnTorque"
  SAPPAngleControlStat6/1(out) -> bus_creator/2  "SAPPAngleControlStat6"
  SAPPAngleControlStat5/1(out) -> bus_creator/3  "SAPPAngleControlStat5"
  SAPPAngleControlStat4/1(out) -> bus_creator/4  "SAPPAngleControlStat4"
  SAPPAngleControlStat3/1(out) -> bus_creator/5  "SAPPAngleControlStat3"
  SAPPAngleControlStat2/1(out) -> bus_creator/6  "SAPPAngleControlStat2"
  DrvSteActv_B_Stat/1(out) -> bus_creator/7  "DrvSteActv_B_Stat"
  EPAS_Failure/1(out) -> bus_creator/8  "EPAS_Failure"
  SAPPAngleControlStat1/1(out) -> bus_creator/9  "SAPPAngleControlStat1"
  SteMdule_I_Est/1(out) -> bus_creator/10  "SteMdule_I_Est"
  VehVTrlrAid_B_Rq/1(out) -> bus_creator/11  "VehVTrlrAid_B_Rq"
  TrlrHitchLamp_D_Rqst/1(out) -> bus_creator/12  "TrlrHitchLamp_D_Rqst"
  SteMdule_U_Meas/1(out) -> bus_creator/13  "SteMdule_U_Meas"
  DrvSte_Tq_Actl/1(out) -> bus_creator/14  "DrvSte_Tq_Actl"
  SteMdule_D_Stat/1(out) -> bus_creator/15  "SteMdule_D_Stat"
  Veh_V_RqMxTrlrAid/1(out) -> bus_creator/16  "Veh_V_RqMxTrlrAid"
  bus_selector/1 -> SteeringColumnTorque/1(in)  "<SteeringColumnTorque>"
  bus_selector/2 -> SAPPAngleControlStat6/1(in)  "<SAPPAngleControlStat6>"
  bus_selector/3 -> SAPPAngleControlStat5/1(in)  "<SAPPAngleControlStat5>"
  bus_selector/4 -> SAPPAngleControlStat4/1(in)  "<SAPPAngleControlStat4>"
  bus_selector/5 -> SAPPAngleControlStat3/1(in)  "<SAPPAngleControlStat3>"
  bus_selector/6 -> SAPPAngleControlStat2/1(in)  "<SAPPAngleControlStat2>"
  bus_selector/7 -> DrvSteActv_B_Stat/1(in)  "<DrvSteActv_B_Stat>"
  bus_selector/8 -> EPAS_Failure/1(in)  "<EPAS_Failure>"
  bus_selector/9 -> SAPPAngleControlStat1/1(in)  "<SAPPAngleControlStat1>"
  bus_selector/10 -> SteMdule_I_Est/1(in)  "<SteMdule_I_Est>"
  bus_selector/11 -> VehVTrlrAid_B_Rq/1(in)  "<VehVTrlrAid_B_Rq>"
  bus_selector/12 -> TrlrHitchLamp_D_Rqst/1(in)  "<TrlrHitchLamp_D_Rqst>"
  bus_selector/13 -> SteMdule_U_Meas/1(in)  "<SteMdule_U_Meas>"
  bus_selector/14 -> DrvSte_Tq_Actl/1(in)  "<DrvSte_Tq_Actl>"
  bus_selector/15 -> SteMdule_D_Stat/1(in)  "<SteMdule_D_Stat>"
  bus_selector/16 -> Veh_V_RqMxTrlrAid/1(in)  "<Veh_V_RqMxTrlrAid>"
  in/1 -> bus_selector/1

== system test_mdl_NI/CAN_Signal/PSCM/Lane_Assist_Data3_FD1_0x3CC ==
  in : Inport
  LaActAvail_D_Actl : Subsystem
  LaActDeny_B_Actl : Subsystem
  LaHandsOff_B_Actl : Subsystem
  LsmcBrkDecelEnbl_D_Rq : Subsystem
  LsmcBrk_Tq_Rq : Subsystem
  TjaHandsOnCnfdnc_B_Est : Subsystem
  TrlrAn_An_TrgtCalc : Subsystem
  bus_creator : BusCreator  Inputs=7
  bus_selector : BusSelector  OutputSignals=LaHandsOff_B_Actl,LaActDeny_B_Actl,LaActAvail_D_Actl,TjaHandsOnCnfdnc_B_Est,LsmcBrkDecelEnbl_D_Rq,LsmcBrk_Tq_Rq,TrlrAn_An_TrgtCalc
  out_port : Outport
  wires:
  bus_creator/1 -> out_port/1  "Lane_Assist_Data3_FD1_0x3CC"
  LaHandsOff_B_Actl/1(out) -> bus_creator/1  "LaHandsOff_B_Actl"
  LaActDeny_B_Actl/1(out) -> bus_creator/2  "LaActDeny_B_Actl"
  LaActAvail_D_Actl/1(out) -> bus_creator/3  "LaActAvail_D_Actl"
  TjaHandsOnCnfdnc_B_Est/1(out) -> bus_creator/4  "TjaHandsOnCnfdnc_B_Est"
  LsmcBrkDecelEnbl_D_Rq/1(out) -> bus_creator/5  "LsmcBrkDecelEnbl_D_Rq"
  LsmcBrk_Tq_Rq/1(out) -> bus_creator/6  "LsmcBrk_Tq_Rq"
  TrlrAn_An_TrgtCalc/1(out) -> bus_creator/7  "TrlrAn_An_TrgtCalc"
  bus_selector/1 -> LaHandsOff_B_Actl/1(in)  "<LaHandsOff_B_Actl>"
  bus_selector/2 -> LaActDeny_B_Actl/1(in)  "<LaActDeny_B_Actl>"
  bus_selector/3 -> LaActAvail_D_Actl/1(in)  "<LaActAvail_D_Actl>"
  bus_selector/4 -> TjaHandsOnCnfdnc_B_Est/1(in)  "<TjaHandsOnCnfdnc_B_Est>"
  bus_selector/5 -> LsmcBrkDecelEnbl_D_Rq/1(in)  "<LsmcBrkDecelEnbl_D_Rq>"
  bus_selector/6 -> LsmcBrk_Tq_Rq/1(in)  "<LsmcBrk_Tq_Rq>"
  bus_selector/7 -> TrlrAn_An_TrgtCalc/1(in)  "<TrlrAn_An_TrgtCalc>"
  in/1 -> bus_selector/1

== system test_mdl_NI/CAN_Signal/PSCM/PSCM_AutoSar_NetwrkMgmt_0x5B5 ==
  in : Inport
  PSCM_AutoSarNMControl : Subsystem
  PSCM_AutoSarNMNodeId : Subsystem
  PSCM_AutoSarNMReserved1 : Subsystem
  PSCM_AutoSarNMReserved2 : Subsystem
  PSCM_AutoSarNMReserved3 : Subsystem
  PSCM_AutoSarNMReserved4 : Subsystem
  PSCM_GWNMProxy : Subsystem
  PSCM_GWOnBoardTester : Subsystem
  bus_creator : BusCreator  Inputs=8
  bus_selector : BusSelector  OutputSignals=PSCM_AutoSarNMNodeId,PSCM_AutoSarNMControl,PSCM_AutoSarNMReserved1,PSCM_AutoSarNMReserved2,PSCM_GWOnBoardTester,PSCM_GWNMProxy,PSCM_AutoSarNMReserved3,PSCM_AutoSarNMReserved4
  out_port : Outport
  wires:
  bus_creator/1 -> out_port/1  "PSCM_AutoSar_NetwrkMgmt_0x5B5"
  PSCM_AutoSarNMNodeId/1(out) -> bus_creator/1  "PSCM_AutoSarNMNodeId"
  PSCM_AutoSarNMControl/1(out) -> bus_creator/2  "PSCM_AutoSarNMControl"
  PSCM_AutoSarNMReserved1/1(out) -> bus_creator/3  "PSCM_AutoSarNMReserved1"
  PSCM_AutoSarNMReserved2/1(out) -> bus_creator/4  "PSCM_AutoSarNMReserved2"
  PSCM_GWOnBoardTester/1(out) -> bus_creator/5  "PSCM_GWOnBoardTester"
  PSCM_GWNMProxy/1(out) -> bus_creator/6  "PSCM_GWNMProxy"
  PSCM_AutoSarNMReserved3/1(out) -> bus_creator/7  "PSCM_AutoSarNMReserved3"
  PSCM_AutoSarNMReserved4/1(out) -> bus_creator/8  "PSCM_AutoSarNMReserved4"
  bus_selector/1 -> PSCM_AutoSarNMNodeId/1(in)  "<PSCM_AutoSarNMNodeId>"
  bus_selector/2 -> PSCM_AutoSarNMControl/1(in)  "<PSCM_AutoSarNMControl>"
  bus_selector/3 -> PSCM_AutoSarNMReserved1/1(in)  "<PSCM_AutoSarNMReserved1>"
  bus_selector/4 -> PSCM_AutoSarNMReserved2/1(in)  "<PSCM_AutoSarNMReserved2>"
  bus_selector/5 -> PSCM_GWOnBoardTester/1(in)  "<PSCM_GWOnBoardTester>"
  bus_selector/6 -> PSCM_GWNMProxy/1(in)  "<PSCM_GWNMProxy>"
  bus_selector/7 -> PSCM_AutoSarNMReserved3/1(in)  "<PSCM_AutoSarNMReserved3>"
  bus_selector/8 -> PSCM_AutoSarNMReserved4/1(in)  "<PSCM_AutoSarNMReserved4>"
  in/1 -> bus_selector/1

== system test_mdl_NI/CAN_Signal/PSCM/SteeringPinion_Data_0x7E ==
  in : Inport
  StePinAn_No_Cnt : Subsystem
  StePinAn_No_Cs : Subsystem
  StePinCompAnEst_D_Qf : Subsystem
  StePinComp_An_Est : Subsystem
  StePinRelInit_An_Sns : Subsystem
  StePw_B_Rq : Subsystem
  bus_creator : BusCreator  Inputs=6
  bus_selector : BusSelector  OutputSignals=StePinRelInit_An_Sns,StePw_B_Rq,StePinComp_An_Est,StePinAn_No_Cs,StePinAn_No_Cnt,StePinCompAnEst_D_Qf
  out_port : Outport
  wires:
  bus_creator/1 -> out_port/1  "SteeringPinion_Data_0x7E"
  StePinRelInit_An_Sns/1(out) -> bus_creator/1  "StePinRelInit_An_Sns"
  StePw_B_Rq/1(out) -> bus_creator/2  "StePw_B_Rq"
  StePinComp_An_Est/1(out) -> bus_creator/3  "StePinComp_An_Est"
  StePinAn_No_Cs/1(out) -> bus_creator/4  "StePinAn_No_Cs"
  StePinAn_No_Cnt/1(out) -> bus_creator/5  "StePinAn_No_Cnt"
  StePinCompAnEst_D_Qf/1(out) -> bus_creator/6  "StePinCompAnEst_D_Qf"
  bus_selector/1 -> StePinRelInit_An_Sns/1(in)  "<StePinRelInit_An_Sns>"
  bus_selector/2 -> StePw_B_Rq/1(in)  "<StePw_B_Rq>"
  bus_selector/3 -> StePinComp_An_Est/1(in)  "<StePinComp_An_Est>"
  bus_selector/4 -> StePinAn_No_Cs/1(in)  "<StePinAn_No_Cs>"
  bus_selector/5 -> StePinAn_No_Cnt/1(in)  "<StePinAn_No_Cnt>"
  bus_selector/6 -> StePinCompAnEst_D_Qf/1(in)  "<StePinCompAnEst_D_Qf>"
  in/1 -> bus_selector/1

== system test_mdl_NI/CAN_Signal/PSCM/TesterPhysicalResPSCM_0x738 ==
  in : Inport
  TesterPhysicalResPSCM : Subsystem
  bus_creator : BusCreator  Inputs=1
  bus_selector : BusSelector  OutputSignals=TesterPhysicalResPSCM
  out_port : Outport
  wires:
  bus_creator/1 -> out_port/1  "TesterPhysicalResPSCM_0x738"
  TesterPhysicalResPSCM/1(out) -> bus_creator/1  "TesterPhysicalResPSCM"
  bus_selector/1 -> TesterPhysicalResPSCM/1(in)  "<TesterPhysicalResPSCM>"
  in/1 -> bus_selector/1

== system test_mdl_NI/CAN_Signal/PSCM/TrailerAid_Data2_0x417 ==
  in : Inport
  EsaOn_B_Stat : Subsystem
  HitchToTrlrAxle_L_Calc : Subsystem
  LatCtlLim_D_Stat : Subsystem
  LatCtlSte_D_Stat : Subsystem
  SelDrvMdeSte_D_Stat : Subsystem
  TrlrAidEnbl_D2_Stat : Subsystem
  TrlrAidMsgTxt_D2_Rq : Subsystem
  TrlrAidSetup_D2_Stat : Subsystem
  TrlrAidTrgtId_No_Rq : Subsystem
  TrlrAidTrlrId_No_Rq : Subsystem
  TrlrAnOffst_An2_Calc : Subsystem
  TrlrAn_An_MxCalc : Subsystem
  TrlrAn_An_WarnCalc : Subsystem
  bus_creator : BusCreator  Inputs=13
  bus_selector : BusSelector  OutputSignals=HitchToTrlrAxle_L_Calc,TrlrAidMsgTxt_D2_Rq,EsaOn_B_Stat,LatCtlLim_D_Stat,LatCtlSte_D_Stat,SelDrvMdeSte_D_Stat,TrlrAidEnbl_D2_Stat,TrlrAn_An_WarnCalc,TrlrAnOffst_An2_Calc,TrlrAidSetup_D2_Stat,TrlrAidTrgtId_No_Rq,TrlrAn_An_MxCalc,TrlrAidTrlrId_No_Rq
  out_port : Outport
  wires:
  bus_creator/1 -> out_port/1  "TrailerAid_Data2_0x417"
  HitchToTrlrAxle_L_Calc/1(out) -> bus_creator/1  "HitchToTrlrAxle_L_Calc"
  TrlrAidMsgTxt_D2_Rq/1(out) -> bus_creator/2  "TrlrAidMsgTxt_D2_Rq"
  EsaOn_B_Stat/1(out) -> bus_creator/3  "EsaOn_B_Stat"
  LatCtlLim_D_Stat/1(out) -> bus_creator/4  "LatCtlLim_D_Stat"
  LatCtlSte_D_Stat/1(out) -> bus_creator/5  "LatCtlSte_D_Stat"
  SelDrvMdeSte_D_Stat/1(out) -> bus_creator/6  "SelDrvMdeSte_D_Stat"
  TrlrAidEnbl_D2_Stat/1(out) -> bus_creator/7  "TrlrAidEnbl_D2_Stat"
  TrlrAn_An_WarnCalc/1(out) -> bus_creator/8  "TrlrAn_An_WarnCalc"
  TrlrAnOffst_An2_Calc/1(out) -> bus_creator/9  "TrlrAnOffst_An2_Calc"
  TrlrAidSetup_D2_Stat/1(out) -> bus_creator/10  "TrlrAidSetup_D2_Stat"
  TrlrAidTrgtId_No_Rq/1(out) -> bus_creator/11  "TrlrAidTrgtId_No_Rq"
  TrlrAn_An_MxCalc/1(out) -> bus_creator/12  "TrlrAn_An_MxCalc"
  TrlrAidTrlrId_No_Rq/1(out) -> bus_creator/13  "TrlrAidTrlrId_No_Rq"
  bus_selector/1 -> HitchToTrlrAxle_L_Calc/1(in)  "<HitchToTrlrAxle_L_Calc>"
  bus_selector/2 -> TrlrAidMsgTxt_D2_Rq/1(in)  "<TrlrAidMsgTxt_D2_Rq>"
  bus_selector/3 -> EsaOn_B_Stat/1(in)  "<EsaOn_B_Stat>"
  bus_selector/4 -> LatCtlLim_D_Stat/1(in)  "<LatCtlLim_D_Stat>"
  bus_selector/5 -> LatCtlSte_D_Stat/1(in)  "<LatCtlSte_D_Stat>"
  bus_selector/6 -> SelDrvMdeSte_D_Stat/1(in)  "<SelDrvMdeSte_D_Stat>"
  bus_selector/7 -> TrlrAidEnbl_D2_Stat/1(in)  "<TrlrAidEnbl_D2_Stat>"
  bus_selector/8 -> TrlrAn_An_WarnCalc/1(in)  "<TrlrAn_An_WarnCalc>"
  bus_selector/9 -> TrlrAnOffst_An2_Calc/1(in)  "<TrlrAnOffst_An2_Calc>"
  bus_selector/10 -> TrlrAidSetup_D2_Stat/1(in)  "<TrlrAidSetup_D2_Stat>"
  bus_selector/11 -> TrlrAidTrgtId_No_Rq/1(in)  "<TrlrAidTrgtId_No_Rq>"
  bus_selector/12 -> TrlrAn_An_MxCalc/1(in)  "<TrlrAn_An_MxCalc>"
  bus_selector/13 -> TrlrAidTrlrId_No_Rq/1(in)  "<TrlrAidTrlrId_No_Rq>"
  in/1 -> bus_selector/1

== system test_mdl_NI/CAN_Signal/RealPCM/EngBrakeData ==
  in : Inport
  CcStat_D_Actl : Subsystem
  bus_creator : BusCreator  Inputs=1
  bus_selector : BusSelector  OutputSignals=CcStat_D_Actl
  out_port : Outport
  wires:
  bus_creator/1 -> out_port/1  "EngBrakeData"
  CcStat_D_Actl/1(out) -> bus_creator/1  "CcStat_D_Actl"
  bus_selector/1 -> CcStat_D_Actl/1(in)  "<CcStat_D_Actl>"
  in/1 -> bus_selector/1

== system test_mdl_NI/CAN_Signal/RealPCM/EngVehicleSpThrottle2 ==
  in : Inport
  Veh_V_ActlEng : Subsystem
  bus_creator : BusCreator  Inputs=1
  bus_selector : BusSelector  OutputSignals=Veh_V_ActlEng
  out_port : Outport
  wires:
  bus_creator/1 -> out_port/1  "EngVehicleSpThrottle2"
  Veh_V_ActlEng/1(out) -> bus_creator/1  "Veh_V_ActlEng"
  bus_selector/1 -> Veh_V_ActlEng/1(in)  "<Veh_V_ActlEng>"
  in/1 -> bus_selector/1

== system test_mdl_NI/CAN_Signal/RealPCM/user_channel ==
  in : Inport
  Desired_Speed : Subsystem
  PCM_status_user_input : Subsystem
  bus_creator : BusCreator  Inputs=2
  bus_selector : BusSelector  OutputSignals=PCM_status_user_input,Desired_Speed
  out_port : Outport
  wires:
  bus_creator/1 -> out_port/1  "user_channel"
  PCM_status_user_input/1(out) -> bus_creator/1  "PCM_status_user_input"
  Desired_Speed/1(out) -> bus_creator/2  "Desired_Speed"
  bus_selector/1 -> PCM_status_user_input/1(in)  "<PCM_status_user_input>"
  bus_selector/2 -> Desired_Speed/1(in)  "<Desired_Speed>"
  in/1 -> bus_selector/1

== system test_mdl_NI/Subsystem/ABS_ESC/ABS_AutoSar_NetworkMgt_Ox596 ==
  in_port : Inport
  ABS_AutoSarNMControl : Terminator
  ABS_AutoSarNMNodeId : Terminator
  ABS_AutoSarNMReserved{1..4} (4 alike) : Terminator
  ABS_GWNMProxy : Terminator
  ABS_GWOnBoardTester : Terminator
  bus_selector : BusSelector  OutputSignals=ABS_AutoSarNMControl,ABS_AutoSarNMNodeId,ABS_AutoSarNMReserved1,ABS_AutoSarNMReserved2,ABS_AutoSarNMReserved3,ABS_AutoSarNMReserved4,ABS_GWNMProxy,ABS_GWOnBoardTester
  wires:
  in_port/1 -> bus_selector/1  "ABS_AutoSar_NetworkMgt_Ox596"
  bus_selector/1 -> ABS_AutoSarNMControl/1  "<ABS_AutoSarNMControl>"
  bus_selector/2 -> ABS_AutoSarNMNodeId/1  "<ABS_AutoSarNMNodeId>"
  bus_selector/3 -> ABS_AutoSarNMReserved1/1  "<ABS_AutoSarNMReserved1>"
  bus_selector/4 -> ABS_AutoSarNMReserved2/1  "<ABS_AutoSarNMReserved2>"
  bus_selector/5 -> ABS_AutoSarNMReserved3/1  "<ABS_AutoSarNMReserved3>"
  bus_selector/6 -> ABS_AutoSarNMReserved4/1  "<ABS_AutoSarNMReserved4>"
  bus_selector/7 -> ABS_GWNMProxy/1  "<ABS_GWNMProxy>"
  bus_selector/8 -> ABS_GWOnBoardTester/1  "<ABS_GWOnBoardTester>"

== system test_mdl_NI/Subsystem/ABS_ESC/ABS_BrkBst_Data_Ox4B0 ==
  in_port : Inport
  BrkBstrVac_P_Actl : Terminator
  BrkHold_D_Stat : Terminator
  BrkTotTqRqDrv_No_Cnt : Terminator
  BrkTotTqRqDrv_No_Cs : Terminator
  BrkTot_Tq_RqDrv : Terminator
  HsaStat_D_Dsply : Terminator
  HsaTrnAout_Tq_Rq : Terminator
  YawStabilityIndex : Terminator
  bus_selector : BusSelector  OutputSignals=BrkBstrVac_P_Actl,BrkHold_D_Stat,BrkTotTqRqDrv_No_Cnt,BrkTotTqRqDrv_No_Cs,BrkTot_Tq_RqDrv,HsaStat_D_Dsply,HsaTrnAout_Tq_Rq,YawStabilityIndex
  wires:
  in_port/1 -> bus_selector/1  "ABS_BrkBst_Data_Ox4B0"
  bus_selector/1 -> BrkBstrVac_P_Actl/1  "<BrkBstrVac_P_Actl>"
  bus_selector/2 -> BrkHold_D_Stat/1  "<BrkHold_D_Stat>"
  bus_selector/3 -> BrkTotTqRqDrv_No_Cnt/1  "<BrkTotTqRqDrv_No_Cnt>"
  bus_selector/4 -> BrkTotTqRqDrv_No_Cs/1  "<BrkTotTqRqDrv_No_Cs>"
  bus_selector/5 -> BrkTot_Tq_RqDrv/1  "<BrkTot_Tq_RqDrv>"
  bus_selector/6 -> HsaStat_D_Dsply/1  "<HsaStat_D_Dsply>"
  bus_selector/7 -> HsaTrnAout_Tq_Rq/1  "<HsaTrnAout_Tq_Rq>"
  bus_selector/8 -> YawStabilityIndex/1  "<YawStabilityIndex>"

== system test_mdl_NI/Subsystem/ABS_ESC/ABS_Rapid_Data_Response_1_Ox6B0 ==
  in_port : Inport
  UUDTABSResponse1 : Terminator
  bus_selector : BusSelector  OutputSignals=UUDTABSResponse1
  wires:
  in_port/1 -> bus_selector/1  "ABS_Rapid_Data_Response_1_Ox6B0"
  bus_selector/1 -> UUDTABSResponse1/1  "<UUDTABSResponse1>"

== system test_mdl_NI/Subsystem/ABS_ESC/ABS_Rapid_Data_Response_2_Ox6B1 ==
  in_port : Inport
  UUDTABSResponse2 : Terminator
  bus_selector : BusSelector  OutputSignals=UUDTABSResponse2
  wires:
  in_port/1 -> bus_selector/1  "ABS_Rapid_Data_Response_2_Ox6B1"
  bus_selector/1 -> UUDTABSResponse2/1  "<UUDTABSResponse2>"

== system test_mdl_NI/Subsystem/ABS_ESC/ActiveFronSteering_Req_Ox88 ==
  in_port : Inport
  SteWhlBrkAnRq_No_Cnt : Terminator
  SteWhlBrkAnRq_No_Cs : Terminator
  SteWhlBrkOffst_An_Rq : Terminator
  bus_selector : BusSelector  OutputSignals=SteWhlBrkAnRq_No_Cnt,SteWhlBrkAnRq_No_Cs,SteWhlBrkOffst_An_Rq
  wires:
  in_port/1 -> bus_selector/1  "ActiveFronSteering_Req_Ox88"
  bus_selector/1 -> SteWhlBrkAnRq_No_Cnt/1  "<SteWhlBrkAnRq_No_Cnt>"
  bus_selector/2 -> SteWhlBrkAnRq_No_Cs/1  "<SteWhlBrkAnRq_No_Cs>"
  bus_selector/3 -> SteWhlBrkOffst_An_Rq/1  "<SteWhlBrkOffst_An_Rq>"

== system test_mdl_NI/Subsystem/ABS_ESC/BrakeSnData_3_Ox77 ==
  in_port : Inport
  VehLatComp_A_Actl : Terminator
  VehLongComp_A_Actl : Terminator
  VehOverGnd_V_Est : Terminator
  VehTrvlDir_D_Stat : Terminator
  VehYawComp_W_Actl : Terminator
  bus_selector : BusSelector  OutputSignals=VehLatComp_A_Actl,VehLongComp_A_Actl,VehOverGnd_V_Est,VehTrvlDir_D_Stat,VehYawComp_W_Actl
  wires:
  in_port/1 -> bus_selector/1  "BrakeSnData_3_Ox77"
  bus_selector/1 -> VehLatComp_A_Actl/1  "<VehLatComp_A_Actl>"
  bus_selector/2 -> VehLongComp_A_Actl/1  "<VehLongComp_A_Actl>"
  bus_selector/3 -> VehOverGnd_V_Est/1  "<VehOverGnd_V_Est>"
  bus_selector/4 -> VehTrvlDir_D_Stat/1  "<VehTrvlDir_D_Stat>"
  bus_selector/5 -> VehYawComp_W_Actl/1  "<VehYawComp_W_Actl>"

== system test_mdl_NI/Subsystem/ABS_ESC/BrakeSnData_4_Ox7D ==
  in_port : Inport
  BrkTotTqRqArb_No_Cnt : Terminator
  BrkTotTqRqArb_No_Cs : Terminator
  BrkTot_Tq_Actl : Terminator
  BrkTot_Tq_RqArb : Terminator
  HsaStat_D_Actl : Terminator
  VehRolComp_W_Actl : Terminator
  VehVertComp_A_Actl : Terminator
  bus_selector : BusSelector  OutputSignals=BrkTotTqRqArb_No_Cnt,BrkTotTqRqArb_No_Cs,BrkTot_Tq_Actl,BrkTot_Tq_RqArb,HsaStat_D_Actl,VehRolComp_W_Actl,VehVertComp_A_Actl
  wires:
  in_port/1 -> bus_selector/1  "BrakeSnData_4_Ox7D"
  bus_selector/1 -> BrkTotTqRqArb_No_Cnt/1  "<BrkTotTqRqArb_No_Cnt>"
  bus_selector/2 -> BrkTotTqRqArb_No_Cs/1  "<BrkTotTqRqArb_No_Cs>"
  bus_selector/3 -> BrkTot_Tq_Actl/1  "<BrkTot_Tq_Actl>"
  bus_selector/4 -> BrkTot_Tq_RqArb/1  "<BrkTot_Tq_RqArb>"
  bus_selector/5 -> HsaStat_D_Actl/1  "<HsaStat_D_Actl>"
  bus_selector/6 -> VehRolComp_W_Actl/1  "<VehRolComp_W_Actl>"
  bus_selector/7 -> VehVertComp_A_Actl/1  "<VehVertComp_A_Actl>"

== system test_mdl_NI/Subsystem/ABS_ESC/BrakeSnData_5_Ox76 ==
  in_port : Inport
  AwdLck_Tq_RqMn : Terminator
  AwdLck_Tq_RqMx : Terminator
  BrkCtrFnd_B_Stat : Terminator
  DrvSte_D_Stat : Terminator
  DrvSte_Tq_Rq : Terminator
  EmgcyBrkLamp_D_Rq : Terminator
  StopLamp_B_RqBrk : Terminator
  bus_selector : BusSelector  OutputSignals=AwdLck_Tq_RqMn,AwdLck_Tq_RqMx,BrkCtrFnd_B_Stat,DrvSte_D_Stat,DrvSte_Tq_Rq,EmgcyBrkLamp_D_Rq,StopLamp_B_RqBrk
  wires:
  in_port/1 -> bus_selector/1  "BrakeSnData_5_Ox76"
  bus_selector/1 -> AwdLck_Tq_RqMn/1  "<AwdLck_Tq_RqMn>"
  bus_selector/2 -> AwdLck_Tq_RqMx/1  "<AwdLck_Tq_RqMx>"
  bus_selector/3 -> BrkCtrFnd_B_Stat/1  "<BrkCtrFnd_B_Stat>"
  bus_selector/4 -> DrvSte_D_Stat/1  "<DrvSte_D_Stat>"
  bus_selector/5 -> DrvSte_Tq_Rq/1  "<DrvSte_Tq_Rq>"
  bus_selector/6 -> EmgcyBrkLamp_D_Rq/1  "<EmgcyBrkLamp_D_Rq>"
  bus_selector/7 -> StopLamp_B_RqBrk/1  "<StopLamp_B_RqBrk>"

== system test_mdl_NI/Subsystem/ABS_ESC/BrakeSnData_6_Ox414 ==
  in_port : Inport
  StePinOffst_An_Est : Terminator
  StePinOffst_D_Stat : Terminator
  StePinOffst_No_Cnt : Terminator
  StePinOffst_No_Cs : Terminator
  bus_selector : BusSelector  OutputSignals=StePinOffst_An_Est,StePinOffst_D_Stat,StePinOffst_No_Cnt,StePinOffst_No_Cs
  wires:
  in_port/1 -> bus_selector/1  "BrakeSnData_6_Ox414"
  bus_selector/1 -> StePinOffst_An_Est/1  "<StePinOffst_An_Est>"
  bus_selector/2 -> StePinOffst_D_Stat/1  "<StePinOffst_D_Stat>"
  bus_selector/3 -> StePinOffst_No_Cnt/1  "<StePinOffst_No_Cnt>"
  bus_selector/4 -> StePinOffst_No_Cs/1  "<StePinOffst_No_Cs>"
